simulink model "finalProjectLQGwithIntegralAction"  (R2015b)
settings: Solver=VariableStepAuto  StartTime=0.0  StopTime=50  RelTol=1e-3
undefined symbols (not defined in the file): A1, B1, C, Continuous, K, l1, l2, M, m1, m2, Time, X0
libraries: ctrlSharedLib x1
settings Model: Creator=Rishabh  LastModifiedBy=rbiyani
settings DataIOCC: LimitDataPoints=off
settings DebuggingCC: AllowSymbolicDim=on
settings ModelReferenceCC: PropagateSignalLabelsOutOfModel=on
settings GRTTargetCC: GeneratePreprocessorConditionals=Disable all

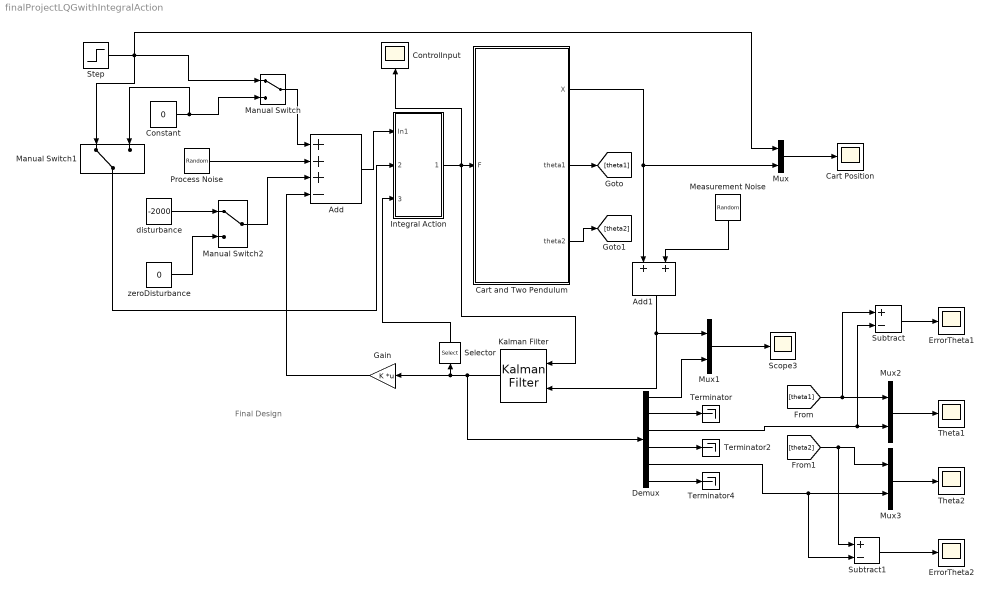
== system finalProjectLQGwithIntegralAction ==
  note: Final Design
  Add : Sum  Inputs=+++-
  Add1 : Sum
  Cart Position : Scope
  "Cart and Two Pendulum " : Subsystem
  Constant : Constant  Value=0
  ControlInput : Scope
  Demux : Demux  Outputs=6
  ErrorTheta1 : Scope
  ErrorTheta2 : Scope
  Gain : Gain  Gain=K  Multiplication=Matrix(K*u)
  Integral Action : Subsystem
  Kalman Filter : ctrlSharedLib/Kalman Filter  TimeDomain=Continuous-Time  UseCurrentEstimator=on  ModelSource=Individual A, B, C, D matrices  ModelSourceVariable=ss(0.95,1,1,0,1)  A=A1  B=B1  C=C  D=0  NumberOfStates=1  NumberOfInputs=1  NumberOfOutputs=1  InitialEstimateSource=Dialog  X0=[2 0 X0(3) 0 X0(5) 0]  P0=10  UseK=off  UseGH=on  NumberOfProcessNoiseInputs=1  G=B1  TimeInvariantG=on  H=0  TimeInvariantH=on  Q=0.2  TimeInvariantQ=on  R=0.001  TimeInvariantR=on  N=0  TimeInvariantN=on  AddInputPort=on  AddEnablePort=off  OutputEstimatedY=off  OutputP=off  Ts=-1
  Manual Switch : ManualSwitch
  Manual Switch1 : ManualSwitch
  Manual Switch2 : ManualSwitch
  Measurement Noise : RandomNumber  Variance=0.001  SampleTime=0.1
  Mux{,1..3} (4 alike) : Mux  Inputs=2
  Process Noise : RandomNumber  Variance=0.2  SampleTime=0.1
  Scope3 : Scope
  Selector : Selector  InputPortWidth=6  IndexOptions=Index vector (dialog)  Indices=[1]  OutputSizes=1
  Step : Step  After=10  SampleTime=0
  Subtract : Sum  Inputs=+-
  Subtract1 : Sum  Inputs=+-
  Terminator : Terminator
  Terminator2 : Terminator
  Terminator4 : Terminator
  Theta1 : Scope
  Theta2 : Scope
  disturbance : Constant  Value=-2000
  zeroDisturbance : Constant  Value=0
  wires:
  "Cart and Two Pendulum "/1(X) -> Mux/2, Add1/1
  Add1/1 -> Mux1/1, Kalman Filter/2
  Kalman Filter/1 -> Selector/1, Gain/1, Demux/1
  Demux/1 -> Mux1/2
  Mux1/1 -> Scope3/1
  Demux/2 -> Terminator/1
  Demux/4 -> Terminator2/1
  Demux/6 -> Terminator4/1
  Demux/3 -> Subtract/2, Mux2/2
  [theta1] -> Subtract/1, Mux2/1
  [theta2] -> Subtract1/1, Mux3/1
  Demux/5 -> Subtract1/2, Mux3/2
  Mux2/1 -> Theta1/1
  Mux3/1 -> Theta2/1
  "Cart and Two Pendulum "/2(theta1) -> [theta1]
  "Cart and Two Pendulum "/3(theta2) -> [theta2]
  Subtract/1 -> ErrorTheta1/1
  Subtract1/1 -> ErrorTheta2/1
  Constant/1 -> Manual Switch1/2, Manual Switch/2
  Manual Switch/1 -> Add/1
  Measurement Noise/1 -> Add1/2
  Process Noise/1 -> Add/2
  Gain/1 -> Add/4
  Step/1 -> Mux/1, Manual Switch1/1, Manual Switch/1
  disturbance/1 -> Manual Switch2/1
  zeroDisturbance/1 -> Manual Switch2/2
  Manual Switch2/1 -> Add/3
  Integral Action/1(Input) -> ControlInput/1, "Cart and Two Pendulum "/1(F), Kalman Filter/1
  Add/1 -> Integral Action/1(In1)
  Manual Switch1/1 -> Integral Action/2(x_ref)
  Selector/1 -> Integral Action/3(x_hat)
  Mux/1 -> Cart Position/1

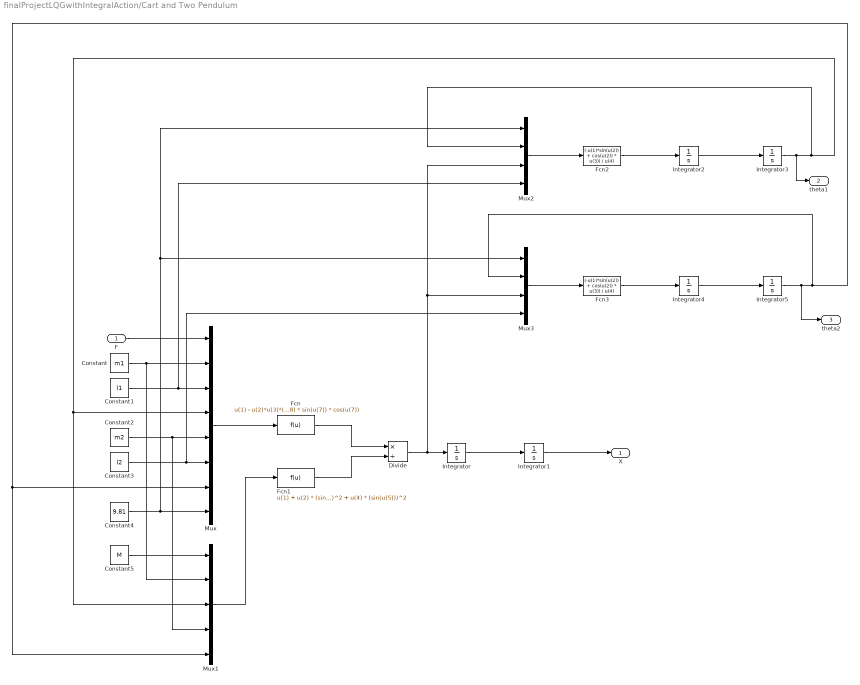
== system finalProjectLQGwithIntegralAction/Cart and Two Pendulum  ==
  F : Inport
  Constant : Constant  Value=m1
  Constant1 : Constant  Value=l1
  Constant2 : Constant  Value=m2
  Constant3 : Constant  Value=l2
  Constant4 : Constant  Value=9.81
  Constant5 : Constant  Value=M
  Divide : Product  Inputs=*/
  Fcn : Fcn  Expr=u(1) - u(2)*u(3)*(u(4)^2)*sin(u(4)) - u(5) * u(6) * (u(7)^2)*sin(u(7))-u(2)*u(8)*sin(u(4))*cos(u(4)) - u(5) * u(8) * sin(u(7)) * cos(u(7))
  Fcn1 : Fcn  Expr=u(1) + u(2) * (sin(u(3)))^2 + u(4) * (sin(u(5)))^2
  Fcn2 : Fcn  Expr=(-u(1)*sin(u(2)) + cos(u(2)) * u(3)) / u(4)
  Fcn3 : Fcn  Expr=(-u(1)*sin(u(2)) + cos(u(2)) * u(3)) / u(4)
  Integrator : Integrator
  Integrator1 : Integrator  InitialCondition=X0(1)
  Integrator2 : Integrator
  Integrator3 : Integrator  InitialCondition=X0(3)
  Integrator4 : Integrator
  Integrator5 : Integrator  InitialCondition=X0(5)
  Mux : Mux  Inputs=8
  Mux1 : Mux  Inputs=5
  Mux2 : Mux
  Mux3 : Mux
  X : Outport
  theta1 : Outport  Port=2
  theta2 : Outport  Port=3
  wires:
  Mux1/1 -> Fcn1/1
  Mux3/1 -> Fcn3/1
  Fcn/1 -> Divide/1
  Integrator2/1 -> Integrator3/1
  Integrator4/1 -> Integrator5/1
  Integrator5/1 -> theta2/1, Mux/7, Mux1/5, Mux3/2
  Integrator3/1 -> theta1/1, Mux2/2, Mux1/3, Mux/4
  Divide/1 -> Mux3/3, Mux2/3, Integrator/1
  Constant5/1 -> Mux1/1
  Constant3/1 -> Mux3/4, Mux/6
  Constant2/1 -> Mux1/4, Mux/5
  Constant/1 -> Mux1/2, Mux/2
  F/1 -> Mux/1
  Constant1/1 -> Mux2/4, Mux/3
  Integrator/1 -> Integrator1/1
  Fcn2/1 -> Integrator2/1
  Constant4/1 -> Mux2/1, Mux3/1, Mux/8
  Mux2/1 -> Fcn2/1
  Integrator1/1 -> X/1
  Mux/1 -> Fcn/1
  Fcn3/1 -> Integrator4/1
  Fcn1/1 -> Divide/2

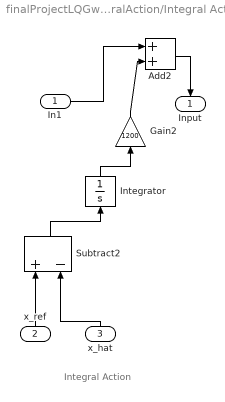
== system finalProjectLQGwithIntegralAction/Integral Action ==
  note: Integral Action
  In1 : Inport
  x_ref : Inport  Port=2
  x_hat : Inport  Port=3
  Add2 : Sum
  Gain2 : Gain  Gain=1200
  Integrator : Integrator
  Subtract2 : Sum  Inputs=+-
  Input : Outport
  wires:
  In1/1 -> Add2/1
  x_hat/1 -> Subtract2/2
  Integrator/1 -> Gain2/1
  Subtract2/1 -> Integrator/1
  Gain2/1 -> Add2/2
  Add2/1 -> Input/1
  x_ref/1 -> Subtract2/1
